simulink model "prelookupTest_2"  (R2017a)
settings: Solver=VariableStepAuto  StartTime=0.0  StopTime=50  RelTol=1e-3
InitFcn:
  | initalize_test
values from neighbouring files (symbols this model uses):
  delta_f = 40    [initalize_test.m]
  deltaCJ = 1    [initalize_test.m]
undefined symbols (not defined in the file or in its folder): cl_fit
libraries: simulink x1
settings Model: Creator=Devansh  LastModifiedBy=Devansh

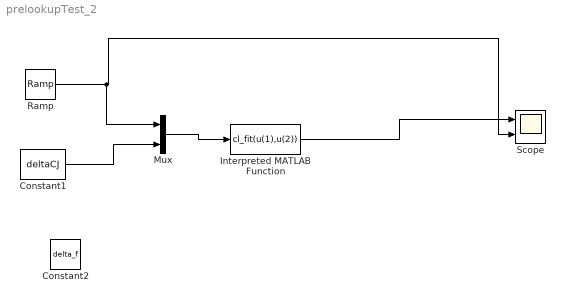
== system prelookupTest_2 ==
  Constant1 : Constant  Value=deltaCJ
  Constant2 : Constant  Value=delta_f
  Interpreted MATLAB Function : MATLABFcn  MATLABFcn=cl_fit(u(1),u(2))  OutputDimensions=1
  Mux : Mux  Inputs=2
  Ramp : simulink/Sources/Ramp  slope=2  start=0  X0=-10
  Scope : Scope  NumInputPorts=2
  wires:
  Interpreted MATLAB Function/1 -> Scope/1
  Ramp/1 -> Mux/1, Scope/2
  Constant1/1 -> Mux/2
  Mux/1 -> Interpreted MATLAB Function/1
